simulink model "motion"  (R2020b)
settings: Solver=VariableStepAuto  StartTime=0.0  StopTime=10.0  RelTol=1e-3
libraries: arduinolib x3, arduinosensorlib x3
settings Model: Creator=gusxo  LastModifiedBy=gusxo

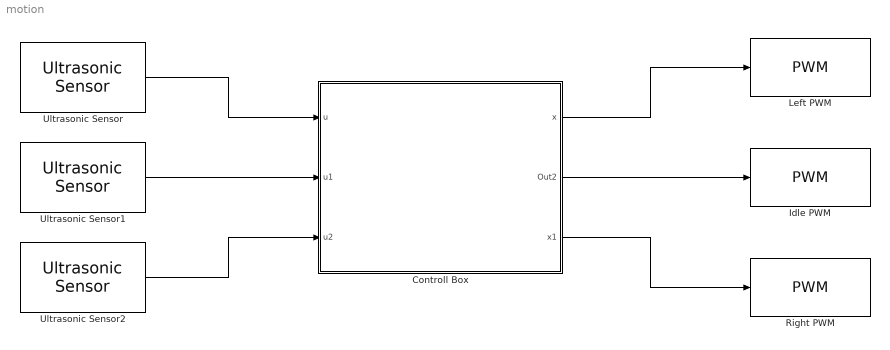
== system motion ==
  Controll Box : Subsystem
  Idle PWM : arduinolib/PWM  pinNumber=5  frequencyType=Default  desiredFrequency=490.2  achievableFrequency=490.2
  Left PWM : arduinolib/PWM  pinNumber=5  frequencyType=Default  desiredFrequency=490.2  achievableFrequency=490.2
  Right PWM : arduinolib/PWM  pinNumber=5  frequencyType=Default  desiredFrequency=490.2  achievableFrequency=490.2
  Ultrasonic Sensor : arduinosensorlib/Ultrasonic Sensor  NumSignalPins=1  TrigPin=4  EchoPin=5  SignalPin=3  SampleTime_=0.1  blockPlatform=ARDUINO
      settings: SourceProductBaseCode=ARDUINO
  Ultrasonic Sensor1 : arduinosensorlib/Ultrasonic Sensor  NumSignalPins=1  TrigPin=4  EchoPin=5  SignalPin=3  SampleTime_=0.1  blockPlatform=ARDUINO
      settings: SourceProductBaseCode=ARDUINO
  Ultrasonic Sensor2 : arduinosensorlib/Ultrasonic Sensor  NumSignalPins=1  TrigPin=4  EchoPin=5  SignalPin=3  SampleTime_=0.1  blockPlatform=ARDUINO
      settings: SourceProductBaseCode=ARDUINO
  wires:
  Ultrasonic Sensor/1 -> Controll Box/1(u)
  Ultrasonic Sensor1/1 -> Controll Box/2(u1)
  Ultrasonic Sensor2/1 -> Controll Box/3(u2)
  Controll Box/1(x) -> Left PWM/1
  Controll Box/2(Out2) -> Idle PWM/1
  Controll Box/3(x1) -> Right PWM/1

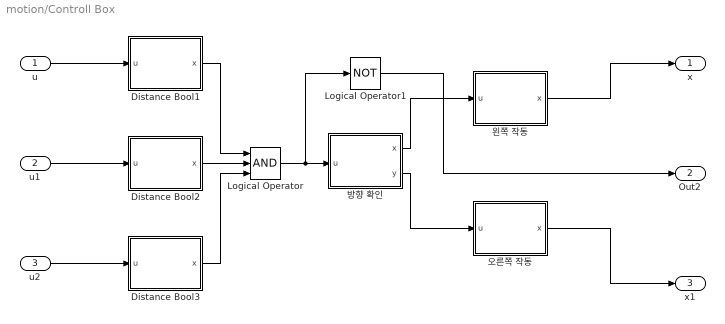
== system motion/Controll Box ==
  u : Inport
  u1 : Inport  Port=2
  u2 : Inport  Port=3
  Distance Bool1 : MATLAB Function  TreatAsAtomicUnit=on
  Distance Bool2 : MATLAB Function  TreatAsAtomicUnit=on
  Distance Bool3 : MATLAB Function  TreatAsAtomicUnit=on
  Logical Operator : Logic  Inputs=3  AllPortsSameDT=off  OutDataTypeStr=boolean
  Logical Operator1 : Logic  Operator=NOT  AllPortsSameDT=off  OutDataTypeStr=boolean
  방향 확인 : MATLAB Function  TreatAsAtomicUnit=on
  오른쪽 작동 : MATLAB Function  TreatAsAtomicUnit=on
  왼쪽 작동 : MATLAB Function  TreatAsAtomicUnit=on
  x : Outport
  Out2 : Outport  Port=2
  x1 : Outport  Port=3
  wires:
  Logical Operator/1 -> Logical Operator1/1, 방향 확인/1(u)
  Distance Bool3/1(x) -> Logical Operator/3
  u2/1 -> Distance Bool3/1(u)
  Distance Bool2/1(x) -> Logical Operator/2
  Distance Bool1/1(x) -> Logical Operator/1
  방향 확인/2(y) -> 오른쪽 작동/1(u)
  u1/1 -> Distance Bool2/1(u)
  u/1 -> Distance Bool1/1(u)
  방향 확인/1(x) -> 왼쪽 작동/1(u)
  오른쪽 작동/1(x) -> x1/1
  왼쪽 작동/1(x) -> x/1
  Logical Operator1/1 -> Out2/1

== matlab function motion/Controll Box/Distance Bool1 ==
  data: u input; x output
function  x = fcn(u)
    u =

== matlab function motion/Controll Box/Distance Bool2 ==
  data: u input; x output
function  x = fcn(u)
    u =

== matlab function motion/Controll Box/방향 확인 ==
  data: u input; x output; y output
function [x,y]= fcn(u)
    u =

== matlab function motion/Controll Box/왼쪽 작동 ==
  data: u input; x output
function  x = fcn(u)
    u =

== matlab function motion/Controll Box/오른쪽 작동 ==
  data: u input; x output
function  x = fcn(u)
    u =

== matlab function motion/Controll Box/Distance Bool3 ==
  data: u input; x output
function  x = fcn(u)
    u =
